simulink model "tp4"  (R2015a)
settings: Solver=ode45  StartTime=0.0  StopTime=0.9  FixedStep=0.01  RelTol=1e-3
values from neighbouring files (symbols this model uses):
  H = 0.144    [fonction.m]    (also in matrices.m)
  K = -place(A,B,V)    [matrices.m]
libraries: simulink x2
settings Model: Creator=fschalle  LastModifiedBy=fschalle

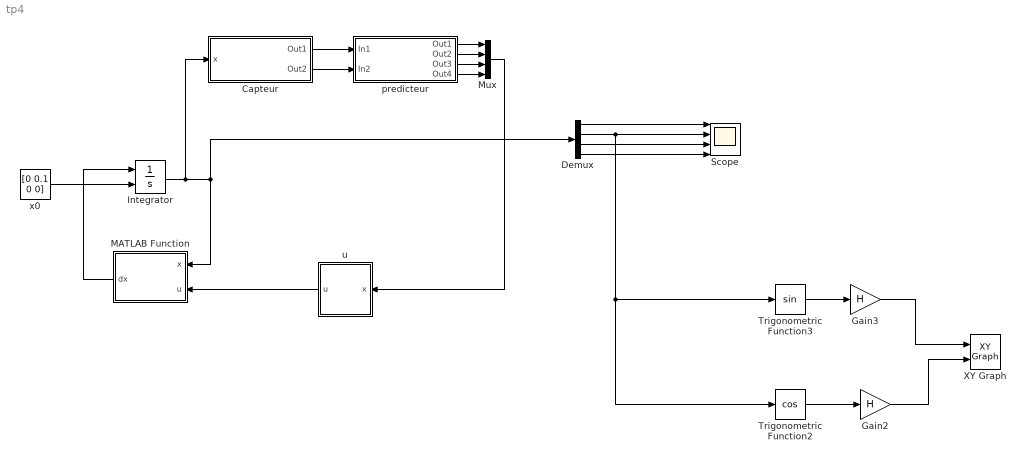
== system tp4 ==
  Capteur : Subsystem  TreatAsAtomicUnit=on
  Demux : Demux
  Gain2 : Gain  Gain=H
  Gain3 : Gain  Gain=H
  Integrator : Integrator  InitialConditionSource=external
  MATLAB Function : MATLAB Function  TreatAsAtomicUnit=on
  Mux : Mux
  Scope : Scope  NumInputPorts=4
      settings: YMin=-15000~-25000~-7e+13~-2.75e+13  YMax=-2000~-5000~4e+13~0
  Trigonometric Function2 : Trigonometry  Operator=cos
  Trigonometric Function3 : Trigonometry
  XY Graph : simulink/Sinks/XY Graph  xmin=-1  xmax=1  ymin=-1  ymax=1  st=-1
  "predicteur " : Subsystem  TreatAsAtomicUnit=on
  "u " : Subsystem
  "x0 " : Constant  Value=[0 0.1 0 0]
  wires:
  MATLAB Function/1(dx) -> Integrator/1
  Integrator/1 -> Capteur/1(x), MATLAB Function/1(x), Demux/1
  "u "/1(u) -> MATLAB Function/2(u)
  Demux/1 -> Scope/1
  Demux/3 -> Scope/3
  Demux/4 -> Scope/4
  "x0 "/1 -> Integrator/2
  Capteur/1(Out1) -> "predicteur "/1(In1)
  Trigonometric Function2/1 -> Gain2/1
  Trigonometric Function3/1 -> Gain3/1
  Gain2/1 -> XY Graph/2
  Gain3/1 -> XY Graph/1
  Demux/2 -> Trigonometric Function3/1, Trigonometric Function2/1, Scope/2
  Capteur/2(Out2) -> "predicteur "/2(In2)
  "predicteur "/1(Out1) -> Mux/1
  "predicteur "/2(Out2) -> Mux/2
  "predicteur "/3(Out3) -> Mux/3
  "predicteur "/4(Out4) -> Mux/4
  Mux/1 -> "u "/1(x)

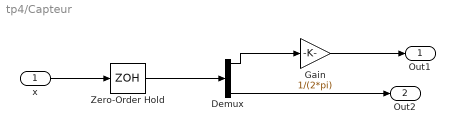
== system tp4/Capteur ==
  x : Inport
  Demux : Demux
  Gain : Gain  Gain=1/(2*pi)
  Zero-Order Hold : ZeroOrderHold
  Out1 : Outport
  Out2 : Outport  Port=2
  wires:
  Demux/4 -> Out2/1
  Gain/1 -> Out1/1
  Demux/1 -> Gain/1
  Zero-Order Hold/1 -> Demux/1
  x/1 -> Zero-Order Hold/1

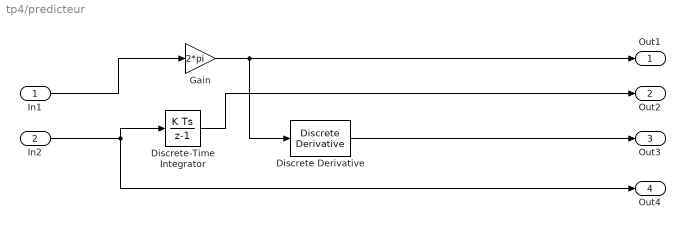
== system tp4/predicteur  ==
  In1 : Inport
  In2 : Inport  Port=2
  Discrete Derivative : simulink/Discrete/Discrete Derivative  gainval=1.0  ICPrevScaledInput=0.0  InputProcessing=Inherited  OutMin=[]  OutMax=[]  OutDataType=fixdt(1, 16)  OutScaling=2^-10  DoSatur=off
  Discrete-Time Integrator : DiscreteIntegrator  InitialConditionSetting=State (most efficient)
  Gain : Gain  Gain=2*pi
  Out1 : Outport
  Out2 : Outport  Port=2
  Out3 : Outport  Port=3
  Out4 : Outport  Port=4
  wires:
  In2/1 -> Discrete-Time Integrator/1, Out4/1
  Discrete-Time Integrator/1 -> Out2/1
  Gain/1 -> Discrete Derivative/1, Out1/1
  In1/1 -> Gain/1
  Discrete Derivative/1 -> Out3/1

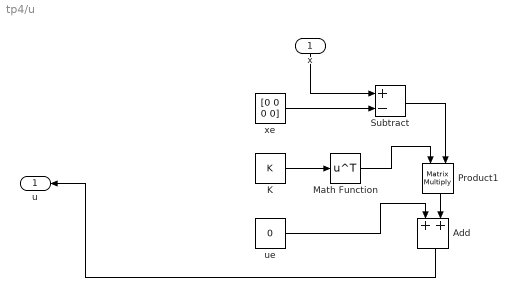
== system tp4/u  ==
  x : Inport
  Add : Sum
  "K " : Constant  Value=K
  Math Function : Math  Operator=transpose  SaturateOnIntegerOverflow=on
  Product1 : Product  Multiplication=Matrix(*)
  Subtract : Sum  Inputs=+-
  ue : Constant  Value=0
  xe : Constant  Value=[0 0 0 0]
  u : Outport
  wires:
  Add/1 -> u/1
  x/1 -> Subtract/1
  ue/1 -> Add/1
  Product1/1 -> Add/2
  Subtract/1 -> Product1/2
  "K "/1 -> Math Function/1
  Math Function/1 -> Product1/1
  xe/1 -> Subtract/2

== matlab function tp4/MATLAB Function ==
  data: x input; u input; dx output
function dx   = fonction( x, u)
%   Dynamic equations of motion of the segway on an axis.
%   Inputs: - x = [theta psi dtheta dpsi]
%               theta: average angle of the wheels      [rad]
%               psi: body pitch angle                   [rad]
%               dtheta: average velocity of the wheels  [rad/s]
%               dpsi: body pitch velocity               [rad/s]
%          - u: DC motor voltage (same value for both motors) [V]

    % State
    psi = x(2);
    dtheta = x(3);
    dpsi = x(4);

    % Parameters
    
    g = 9.81;           % gravity acceleration [m/sec^2]
    m = 0.03;           % wheel weight [kg]
    R = 0.04;           % wheel radius [m]
    Jw = m*R^2/2;       % wheel inertia moment [kg*m^2]
    M = 0.6;            % body weight [kg]
    H = 0.144;          % body height [m]
    L = H/2;            % distance of the center of mass from the wheel axle [m]
    Jpsi = M*L^2/3;     % body pitch inertia [kgm^2]
    Jm = 1e-5;          % DC motor inertia moment [kgm^2]
    Rm = 6.69;          % DC motor resistance [Ohm]
    Kb = 0.468;         % DC motor back EMF constant [Vsec/rad]
    Kt = 0.317;         % DC motor torque constant [Nm/A]
    n = 1;              % gear ratio
    fm = 0.0022;        % friction coefficient between body and DC motor
    fw = 0;             % friction coefficient between wheel and floor
    
    % Equations of motion
    c1 = (2*m+M)*R^2 + 2*Jw + 2*n^2*Jm;
    c2 = M*L*R*cos(psi) - 2*n^2*Jm;
    c3 = -M*L*R*dpsi^2*sin(psi);
    c4 = M*L^2 + Jpsi + 2*n^2*Jm;
    c5 = -M*g*L*sin(psi);

    alpha = Kt/Rm;
    beta = Kt*Kb/Rm + fm;

    Ftheta = alpha*(2*u) - 2*(beta+fw)*dtheta + 2*beta*dpsi;
    Fpsi = -alpha*(2*u) + 2*beta*dtheta - 2*beta*dpsi;

    ddtheta = (c4*c3 - c2*c5 + c4*Ftheta - c2*Fpsi)/(c4*c1 - c2^2);
    ddpsi = (Fpsi- c2*ddtheta - c5)/c4;
    dx = [dtheta dpsi ddtheta ddpsi]';

end
